simulink model "pid_controller1"  (R2014a)
settings: Solver=FixedStepDiscrete  StartTime=0.0  StopTime=10.0  FixedStep=Ts  RelTol=1e-3
undefined symbols (not defined in the file): Fs, Kd, Ki, Kp, Ts
CloseFcn:
  | rtwprivate ssgencode ModelCloseRequest pid_controller
settings Model: BufferReuse=off  Creator=y_yama  LastModifiedBy=yoshi12
settings DataIOCC: SignalLoggingSaveFormat=ModelDataLogs
settings OptimizationCC: BlockReduction=off  InlineParams=on  OptimizeBlockIOStorage=off  BufferReuse=off  GlobalBufferReuse=off  ExpressionFolding=off  ExpressionDepthLimit=2147483647  LocalBlockOutputs=off  InitFltsAndDblsToZero=on  OptimizeModelRefInitCode=on  LifeSpan=1
settings DebuggingCC: SaveWithParameterizedLinksMsg=none  UnderspecifiedInitializationDetection=Classic  SignalResolutionControl=TryResolveAllWithWarning  FcnCallInpInsideContextMsg=UseLocalSettings  StateNameClashWarn=warning
settings HardwareCC: ProdIntDivRoundTo=Zero  ProdEndianess=LittleEndian  ProdHWDeviceType=Intel->x86/Pentium
settings RTWCC: SystemTargetFile=ert.tlc  GenCodeOnly=on  TemplateMakefile=ert_default_tmf  Description=Embedded Coder  GenerateReport=on  ProcessScript=ert_make_rtw_hook  IncludeHyperlinkInReport=on  LaunchReport=on  GenerateTraceInfo=on  GenerateTraceReport=on  GenerateTraceReportSl=on  GenerateTraceReportSf=on  GenerateTraceReportEml=on
settings CodeAppCC: IgnoreCustomStorageClasses=off  CustomSymbolStrType=$N$R$M  InternalIdentifier=Classic
settings ERTTargetCC: ParMdlRefBuildCompliant=on  CompOptLevelCompliant=on  ConcurrentExecutionCompliant=on  ERTFirstTimeCompliant=on  ModelStepFunctionPrototypeControlCompliant=on  CPPClassGenCompliant=on  ERTCustomFileTemplate=example_file_process.tlc

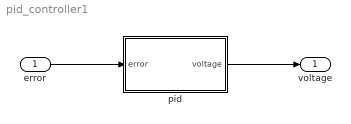
== system pid_controller1 ==
  error : Inport  OutDataTypeStr=single  PortDimensions=1  SampleTime=Ts
      settings: AttributesFormatString=<tsample = %<SampleTime>>
  pid : Subsystem
  voltage : Outport  OutDataTypeStr=single
  wires:
  pid/1(voltage) -> voltage/1
  error/1 -> pid/1(error)

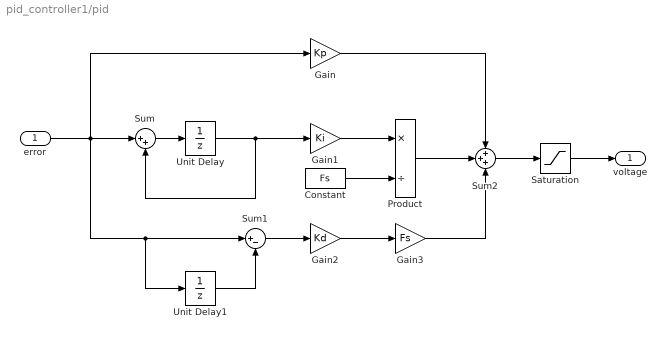
== system pid_controller1/pid ==
  error : Inport
  Constant : Constant  Value=Fs  SampleTime=Ts
  Gain : Gain  Gain=Kp  OutDataTypeStr=Inherit: Same as input
  Gain1 : Gain  Gain=Ki  OutDataTypeStr=Inherit: Same as input
  Gain2 : Gain  Gain=Kd  OutDataTypeStr=Inherit: Same as input
  Gain3 : Gain  Gain=Fs  OutDataTypeStr=Inherit: Same as input
  Product : Product  Inputs=*/  RndMeth=Zero  OutDataTypeStr=Inherit: Same as first input
  Saturation : Saturate  UpperLimit=5  LowerLimit=-5
      settings: AttributesFormatString=<limits = %<UpperLimit> / %<LowerLimit>>
  Sum : Sum  Inputs=|++  OutDataTypeStr=Inherit: Same as first input
  Sum1 : Sum  Inputs=|+-  OutDataTypeStr=Inherit: Same as first input
  Sum2 : Sum  Inputs=+++  OutDataTypeStr=Inherit: Same as first input
  Unit Delay : UnitDelay  SampleTime=-1
      settings: AttributesFormatString=<identifer = %<StateIdentifier>>\n<initial = %<X0>>\n<tsample = %<SampleTime>>
  Unit Delay1 : UnitDelay  SampleTime=-1
      settings: AttributesFormatString=<identifer = %<StateIdentifier>>\n<initial = %<X0>>\n<tsample = %<SampleTime>>
  voltage : Outport
  wires:
  error/1 -> Gain/1, Sum/1, Sum1/1, Unit Delay1/1
  Sum/1 -> Unit Delay/1
  Unit Delay/1 -> Gain1/1, Sum/2
  Gain/1 -> Sum2/1
  Unit Delay1/1 -> Sum1/2
  Sum1/1 -> Gain2/1
  Sum2/1 -> Saturation/1
  Saturation/1 -> voltage/1
  Gain2/1 -> Gain3/1
  Gain1/1 -> Product/1
  Constant/1 -> Product/2
  Product/1 -> Sum2/2
  Gain3/1 -> Sum2/3
